simulink model "Converter4"  (R2025a)
settings: Solver=VariableStepAuto  StartTime=0.0  StopTime=10  MaxStep=1e-3  RelTol=1e-3  EnableMultiTasking=on
PreLoadFcn:
  | DualActiveBridgeConverterData
values from neighbouring files (symbols this model uses):
  C_HV = 100e-6    (= 0.0001)    [Converter_Data.m]
  C_LV = 2000e-6    (= 0.002)    [Converter_Data.m]
  Cs_FET = inf    [Converter_Data.m]
  Fsw = 100e3    (= 100000)    [Converter_Data.m]
  Ki_Ireg = 1    [Converter_Data.m]
  Kp_Ireg = 0.01    [Converter_Data.m]
  L_Inductor = 15e-6    (= 1.5e-05)    [Converter_Data.m]
  Lm_Tr = 720e-6    (= 0.00072)    [Converter_Data.m]
  Lprim_Tr = 17e-6    (= 1.7e-05)    [Converter_Data.m]
  Lsec_Tr = 0    [Converter_Data.m]
  N_Tr = 16    [Converter_Data.m]
  Pnom = 100e3    (= 100000)    [Converter_Data.m]
  R_DCsrc1 = 10e-4    (= 0.001)    [Converter_Data.m]
  R_DCsrc2 = 10e-4    (= 0.001)    [Converter_Data.m]
  R_Inductor = 16e-3    (= 0.016)    [Converter_Data.m]
  RC_HV = 1e-6    (= 1e-06)    [Converter_Data.m]
  RC_LV = 1e-6    (= 1e-06)    [Converter_Data.m]
  Rm_Tr = 10e3    (= 10000)    [Converter_Data.m]
  Ron_Diode = 10e-3    (= 0.01)    [Converter_Data.m]
  Ron_FET = 16e-3    (= 0.016)    [Converter_Data.m]
  Rprim_Tr = 43e-6    (= 4.3e-05)    [Converter_Data.m]
  Rs_FET = 1e6    (= 1000000)    [Converter_Data.m]
  Rsec_Tr = 1e-6    (= 1e-06)    [Converter_Data.m]
  Ts = 1e-6    (= 1e-06)    [Converter_Data.m]
  Ts_Control = Ts    (= 1e-06)    [Converter_Data.m]
  Vf_Diode = 4.2    [Converter_Data.m]
  Vnom_HV = 800    [Converter_Data.m]
  Vnom_LV = 48    [Converter_Data.m]
undefined symbols (not defined in the file or in its folder): DiscIntNeverNeededParam, Ts_Power
libraries: simulink x10, spsDiodeLib x8, spsIdealSwitchLib x8, spsSeriesRLCBranchLib x5, spsVoltageMeasurementLib x4, spsCurrentMeasurementLib x3, spsDCVoltageSourceLib x2, spsMeanLib x2, simulink_extras x2, spsSawtoothGeneratorLib x2, spsFirstOrderFilterLib x1, slpidlib x1
settings Model: ExtModeAutoUpdateStatusClock=off  Creator=The MathWorks, Inc.
settings SolverCC: AlgebraicLoopSolver=TrustRegion  AutoInsertRateTranBlk=on
settings DataIOCC: LimitDataPoints=on  SaveFormat=Array  SaveOutput=off  DSMLogging=off  SaveTime=off  ReturnWorkspaceOutputs=off
settings OptimizationCC: LifeSpan=inf
settings DebuggingCC: SaveWithParameterizedLinksMsg=none  UnderspecifiedInitializationDetection=Classic  MergeDetectMultiDrivingBlocksExec=none  SolverPrmCheckMsg=warning  FcnCallInpInsideContextMsg=warning  UnconnectedInputMsg=warning  UnconnectedOutputMsg=warning  UnconnectedLineMsg=warning  StateNameClashWarn=warning  SubsystemReferenceDiagnosticForUnitTest=warning  SFUnexpectedBacktrackingDiag=warning  SFNoUnconditionalDefaultTransitionDiag=warning  SFExecutionAtInitializationDiag=none  ArithmeticOperatorsInVariantConditions=warning
settings HardwareCC: ProdBitPerPointer=32.0  ProdBitPerSizeT=32.0  ProdBitPerPtrDiffT=32.0  ProdLargestAtomicFloat=None  ProdIntDivRoundTo=Undefined  ProdEndianess=Unspecified  ProdWordSize=32.0  ProdHWDeviceType=32-bit Generic  TargetHWDeviceType=32-bit Generic
settings ModelReferenceCC: EnableRefExpFcnMdlSchedulingChecks=on  PropagateSignalLabelsOutOfModel=off
settings SFSimCC: SimUseLocalCustomCode=off  CustomCodeUndefinedFunction=UseInterfaceOnly
settings RTWCC: RTWUseLocalCustomCode=off  GPUComputeCapability=3.5  DLArmComputeVersion=19.05
settings CodeAppCC: StateflowObjectComments=on
settings GRTTargetCC: TargetFcnLib=ansi_tfl_tmw.mat  TargetLangStandard=C89/C90 (ANSI)  CombineOutputUpdateFcns=off  GRTInterface=on
settings ConfigComp: CovMetricSettings=dw  CovSaveCumulativeToWorkspaceVar=on  CovSaveSingleToWorkspaceVar=on  CovExternalEMLEnable=off  CovSFcnEnable=off

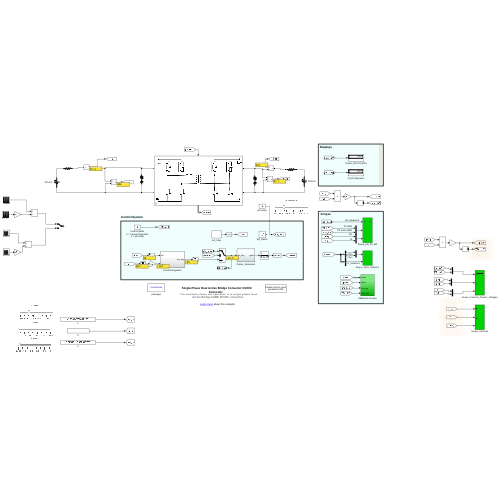
[thumbnail: Simulink's stored preview of the top-level diagram]
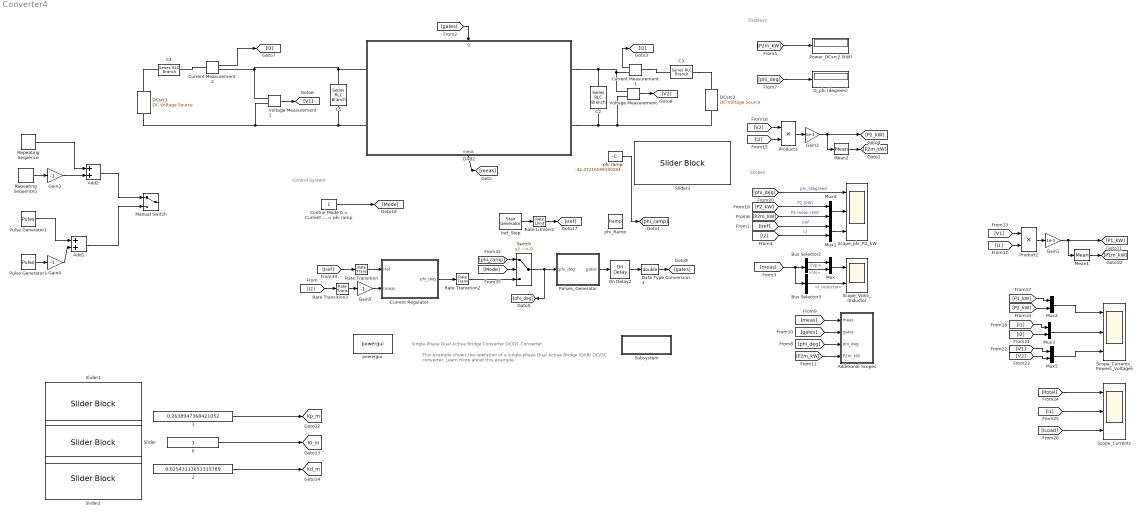
== system Converter4 ==
  note: Single-Phase Dual Active Bridge Converter DC/DC Converter
  note: This example shows the operation of a single-phase Dual Active Bridge (DAB) DC/DC converter.
      |
      | Learn more about this example.
  note: Displays
  note: Scopes
  note: Control System
  0 : Constant
  1 : Constant  Value=0.2638947368421052
  2 : Constant  Value=0.02543113651315789
  Add1 : Sum
  Add2 : Sum
  Additional Scopes : Subsystem
  Bus Selector2 : BusSelector  OutputSignals=Vp,Vs
  Bus Selector3 : BusSelector  OutputSignals=I_Inductor
  C2 : spsSeriesRLCBranchLib/Series RLC Branch  LConnTagsString=__new0  RConnTagsString=__new0  BranchType=RC  Resistance=RC_LV  Inductance=1  SetiL0=off  InitialCurrent=0  Capacitance=C_LV  Setx0=off  InitialVoltage=0  Measurements=None
  C3 : spsSeriesRLCBranchLib/Series RLC Branch  LConnTagsString=__new0  RConnTagsString=__new0  BranchType=R  Resistance=R_DCsrc2  Inductance=100e-6  SetiL0=off  InitialCurrent=0  Capacitance=1  Setx0=off  InitialVoltage=0  Measurements=None
  C4 : spsSeriesRLCBranchLib/Series RLC Branch  LConnTagsString=__new0  RConnTagsString=__new0  BranchType=R  Resistance=R_DCsrc1  Inductance=1  SetiL0=off  InitialCurrent=0  Capacitance=1  Setx0=off  InitialVoltage=0  Measurements=None
  C5 : spsSeriesRLCBranchLib/Series RLC Branch  LConnTagsString=__new0  RConnTagsString=__new0  BranchType=RC  Resistance=RC_HV  Inductance=1  SetiL0=off  InitialCurrent=0  Capacitance=C_HV  Setx0=off  InitialVoltage=0  Measurements=None
  Control Mode 0 = Current Regulator 1 = phi ramp : Constant
  Current Measurement1 : spsCurrentMeasurementLib/Current Measurement  PhasorSimulation=off  OutputType=Complex  PSBequivalent=0
  Current Measurement2 : spsCurrentMeasurementLib/Current Measurement  PhasorSimulation=off  OutputType=Complex  PSBequivalent=0
  Current Regulator : Subsystem
  DAB2 : Subsystem  mask(Single-phase, Dual-Active Bridge DC/DC Converter){Ron_FET=Ron_FET, RsCs_FET=[Rs_FET, Cs_FET], Ron_Diode=Ron_Diode, Vf_Diode=Vf_Diode, RL_Inductor=[R_Inductor, L_Inductor], Param1_Tr=[Pnom, Fsw], Param2_Tr=[Vnom_HV, Rprim_Tr, Lprim_Tr], Param3_Tr=[Vnom_HV/N_Tr, Rsec_Tr, Lsec_Tr], Param4_Tr=[Rm_Tr, Lm_Tr]}
      mask prompts: Ron_FET "Ron FET"; RsCs_FET "FET snubber: [Rs (ohm)  Cs (F)]"; RL_Inductor "Coupling inductor [ R (ohms)   L (H)]"; Param1_Tr "Nominal power and frequency [Pn(VA) fn(Hz)]:"; Param2_Tr "Winding 1 parameters [V1(Vrms) R1(ohm) L1(H)]:"; Param3_Tr "Winding 2 parameters [V2(Vrms) R2(ohm) L2(H)]:"; Param4_Tr "Magnetization resistance and inductance [Rm(ohm) Lm(H)]:"
      mask init:
      | Rs_FET=RsCs_FET(1);
      | Cs_FET=RsCs_FET(2);
      | R_Inductor=RL_Inductor(1);
      | L_Inductor=RL_Inductor(2);
      settings: PortSchema="{\"entries\":[{\"content\":{\"sides\":[{\"content\":{\"connectorIds\":[\"LConn1\",\"LConn2\"]},\"type\":\"ConnectorPlacement.EquallySpacedRectSide\",\"uuid\":\"9324ea44-499c-4ecb-9e49-362befe9c555\"},{\"content\":{\"connectorIds\":[\"RConn1\",\"RConn2\"],\"side\":\"RIGHT\"},\"type\":\"ConnectorPlacement.EquallySpacedRectSide\",\"uuid\":\"1d2d188e-4a2f-457a-9d2e-cac68811a3aa\"},{\"content\":{\"connectorIds\":[\"In1\"],\"side\":\"TOP\"},\"type\":\"ConnectorPlacement.EquallySpacedRectSide\",\"uuid\":\"7f41b21e-a624-46b0-bf38-abdafc8e74d0\"},{\"content\":{\"connectorIds\":[\"Out1\"],\"side\":\"BOTTOM\"},\"type\":\"ConnectorPlacement.EquallySpacedRectSide\",\"uuid\":\"ef27d855-3875-49de-80dc-d9576eabadca\"}]},\"type\":\"ConnectorPlacement.EquallySpacedConnector\",\"uuid\":\"30393c4b-568d-4140-9cdd-d3267fa7bc9d\"}],\"packageUris\":[\"http://schema.mathworks.com/mf0/Connector/R2020b\"],\"version\":\"1.0\"}"
      mask Display: image('DAB_FB1_1.png');
  DCsrc1 : spsDCVoltageSourceLib/DC Voltage Source  Amplitude=Vnom_HV  Measurements=None
  DCsrc2 : spsDCVoltageSourceLib/DC Voltage Source  Amplitude=Vnom_LV  Measurements=None
  D_phi (degrees) : Display
      settings: Format=bank  Decimation=100
  Data Type Conversion1 : DataTypeConversion  OutDataTypeStr=double  SaturateOnIntegerOverflow=off  RndMeth=Floor
  Gain1 : Gain  Gain=1e-3
  Gain2 : Gain  Gain=1e-3
  Gain3 : Gain  Gain=-1
  Gain4 : Gain  Gain=-1
  Gain5 : Gain  Gain=-1
  Iref_Step : spsStairGeneratorLib/Stair Generator  t=[0, 0.01]  e=[0 40]  Ts=0
  Manual Switch : ManualSwitch
  Mean1 : spsMeanLib/Mean  Freq=Fsw  Vinit=0  Ts=0
  Mean2 : spsMeanLib/Mean  Freq=Fsw  Vinit=0  Ts=0
  Mux{,1..5} (6 alike) : Mux  Inputs=2
  On Delay2 : spsOnDelayLib/On Delay  DelayType=On delay  delay=DT  ic=0  Ts=0
  Power_DCsrc2 (kW) : Display
      settings: Format=bank  Decimation=100
  Product1 : Product
  Product2 : Product
  Pulse Generator1 : DiscretePulseGenerator  PulseType=Time based  Amplitude=50  Period=0.5  PulseWidth=50
  Pulse Generator3 : DiscretePulseGenerator  PulseType=Time based  Amplitude=50  Period=0.5  PulseWidth=50  PhaseDelay=0.25
  Pulses_Generator : Subsystem
  Rate Limiter2 : RateLimiter  RisingSlewLimit=3000  FallingSlewLimit=-3000  SampleTimeMode=inherited
  Rate Transition : RateTransition  OutPortSampleTime=Ts_Control
  Rate Transition2 : RateTransition  OutPortSampleTime=0
  Rate Transition3 : RateTransition  OutPortSampleTime=Ts_Control
  Repeating Sequence : simulink/Sources/Repeating Sequence  rep_seq_t=[0 0.25 0.5 0.75 1 ]  rep_seq_y=[0 20 0 0 0]
  Repeating Sequence1 : simulink/Sources/Repeating Sequence  rep_seq_t=[0 0.25 0.5 0.75 1 ]  rep_seq_y=[0 0 0 20 0]
  Scope_Currents : Scope  NumInputPorts=3
      settings: ActiveDisplayYMinimum=-4.638762576316565  ActiveDisplayYMaximum=13.65424069845692  DataLoggingDecimation=Scope_Decimation  DataLoggingVariableName=ScopeData_phi_P2_kW2
  Scope_Currents_Powers_Voltages : Scope  NumInputPorts=3
      settings: ActiveDisplayYMinimum=-39.981992258178039  ActiveDisplayYMaximum=11.99262168602651  DataLoggingDecimation=Scope_Decimation  DataLoggingVariableName=ScopeData_phi_P2_kW1
  Scope_VpVs_IInductor : Scope  NumInputPorts=2
      settings: TimeSpan=0.0001  ActiveDisplayYMinimum=-1012.21746  ActiveDisplayYMaximum=1013.17909  DataLoggingDecimation=Scope_Decimation  DataLoggingVariableName=Scope_VpVs_IInductor
  Scope_phi_P2_kW : Scope  NumInputPorts=3
      settings: ActiveDisplayYMinimum=-12.508064705091812  ActiveDisplayYMaximum=29.1675627450102  DataLoggingDecimation=Scope_Decimation  DataLoggingVariableName=ScopeData_phi_P2_kW
  Slider : SliderBlock  ScaleMin=1  ScaleMax=1000
  Slider1 : SliderBlock  ScaleMin=0.001  ScaleMax=1
  Slider2 : SliderBlock  ScaleMin=1e-06  ScaleMax=1
  Slider3 : SliderBlock  ScaleMin=-90  ScaleMax=90
  Subsystem : Subsystem
      settings: OpenFcn=open('DualActiveBridgeConverterData')
      mask Display: disp('Double-click to open\nparameters file')
  Switch : Switch  Criteria=u2 ~= 0  SaturateOnIntegerOverflow=off  InputSameDT=off
  Voltage Measurement : spsVoltageMeasurementLib/Voltage Measurement  PhasorSimulation=off  OutputType=Complex  PSBequivalent=0
  Voltage Measurement1 : spsVoltageMeasurementLib/Voltage Measurement  PhasorSimulation=off  OutputType=Complex  PSBequivalent=0
  phi ramp : Constant  Value=-42.47216599190284
  phi_Ramp : simulink/Sources/Ramp  slope=200*1/0.04  start=0  InitialOutput=-100
  powergui : spspowerguiLib/powergui  Priority=1  SimulationMode=Continuous  SampleTime=Ts_Power  frequency=60  Iterations=50  frequencyindice=0  Pbase=100e6  ErrMax=1e-4  UnitsV=kV  UnitsW=MW  buscounter=0  FunctionMessages=off  echomessages=off  EnableUseOfTLC=off  CurrentSourceSwitches=on  DisableSnubberDevices=off  DisableRonSwitches=off  DisableVfSwitches=off  DisplayEquations=off  AutomaticDiscreteSolvers=off  SolverType=Tustin/Backward Euler (TBE)  Interpol=off  ExternalGateDelay=off  methode=off  Ts=10  x0status=blocks  SPID=on  SwTol=0  HookPort=off  NonlinearTolerance=1e-4  nMaxIteration=100  ContinueOnMaxIteration=off  RestoreLinks=warning  ResistiveCurrentMeasurement=off  Frange=[0:2:500]  Ylog=off  Xlog=on  ShowGrid=off  save=off  variable=ZData  structure=0  ZoomFFT=off  StartTime=0.0  cycles=1  DisplayStyle=1  fundamental=60  FreqAxis=off  MaxFrequency=1000  frequencyindicesteady=1  RmsSteady=1  display=off
  tag scope: Kd_m=global, Ki_m=global, Kp_m=global
  wires:
  Mean1/1 -> [P1m_kW]
  Gain1/1 -> Mean1/1, [P1_kW]
  [I1] -> Product2/2
  Product2/1 -> Gain1/1
  [V1] -> Product2/1
  [P1_kW] -> Mux2/1
  [P2_kW] -> Mux2/2
  [I1] -> Mux3/1
  [I2] -> Mux3/2
  [V1] -> Mux5/1
  [V2] -> Mux5/2
  Mux2/1 -> Scope_Currents_Powers_Voltages/1
  Mux3/1 -> Scope_Currents_Powers_Voltages/2
  Mux5/1 -> Scope_Currents_Powers_Voltages/3
  Add2/1 -> Manual Switch/1
  Pulse Generator1/1 -> Add1/1
  Gain4/1 -> Add1/2
  Repeating Sequence/1 -> Add2/1
  Pulse Generator3/1 -> Gain4/1
  Gain3/1 -> Add2/2
  Repeating Sequence1/1 -> Gain3/1
  Add1/1 -> Manual Switch/2
  [Itotal] -> Scope_Currents/1
  [I1] -> Scope_Currents/2
  [ILoad] -> Scope_Currents/3
  Product1/1 -> Gain2/1
  Rate Limiter2/1 -> [Iref]
  Pulses_Generator/1(gates) -> On Delay2/1
  Bus Selector2/1 -> Mux/1  "<Vp>"
  [phi_deg] -> Additional Scopes/3(phi_deg)
  [meas] -> Bus Selector3/1, Bus Selector2/1
  Switch/1 -> [phi_deg], Pulses_Generator/1(phi_deg)
  Mux4/1 -> Scope_phi_P2_kW/2
  [phi_deg] -> D_phi (degrees)/1
  Data Type Conversion1/1 -> [gates]
  [P2m_kW] -> Additional Scopes/4(P2m_kW)
  [phi_deg] -> Scope_phi_P2_kW/1  "phi_(degrees)"
  [I2] -> Product1/2
  [Iref] -> Mux1/1  "Iref"
  On Delay2/1 -> Data Type Conversion1/1
  DAB2/1(meas) -> [meas]
  Mux/1 -> Scope_VpVs_IInductor/1
  [P2m_kW] -> Power_DCsrc2 (kW)/1
  Iref_Step/1 -> Rate Limiter2/1
  Current Measurement1/1 -> [I2]
  Gain5/1 -> Current Regulator/2(Imeas)
  Rate Transition2/1 -> Switch/3
  Bus Selector3/1 -> Scope_VpVs_IInductor/2  "<I_Inductor>"
  Bus Selector2/2 -> Mux/2  "<Vs>"
  [V2] -> Product1/1
  [Mode] -> Switch/2
  [Iref] -> Rate Transition/1
  Control Mode 0 = Current Regulator 1 = phi ramp/1 -> [Mode]
  [gates] -> DAB2/1(g)
  Mux1/1 -> Scope_phi_P2_kW/3
  Rate Transition/1 -> Current Regulator/1(Iref)
  phi ramp/1 -> [phi_ramp]
  [I2] -> Rate Transition3/1
  [P2_kW] -> Mux4/1  "P2 (kW)"
  Voltage Measurement/1 -> [V2]
  [gates] -> Additional Scopes/2(gates)
  [phi_ramp] -> Switch/1
  [P2m_kW] -> Mux4/2  "P2 mean (kW)"
  [I2] -> Mux1/2  "I2"
  Gain2/1 -> Mean2/1, [P2_kW]
  [meas] -> Additional Scopes/1(meas)
  Current Regulator/1(phi_deg) -> Rate Transition2/1
  Mean2/1 -> [P2m_kW]
  Voltage Measurement1/1 -> [V1]
  Current Measurement2/1 -> [I1]
  1/1 -> [Kp_m]
  0/1 -> [Ki_m]
  2/1 -> [Kd_m]
  Rate Transition3/1 -> Gain5/1
  connections:
  DCsrc2/LConn1 -- C2/RConn1 -- DAB2/RConn2 -- Voltage Measurement/LConn2
  C5/LConn1 -- Current Measurement2/RConn1 -- Voltage Measurement1/LConn1 -- DAB2/LConn1
  DAB2/LConn2 -- C5/RConn1 -- Voltage Measurement1/LConn2 -- DCsrc1/LConn1
  C2/LConn1 -- Current Measurement1/RConn1 -- Voltage Measurement/LConn1 -- DAB2/RConn1
  C4/RConn1 -- DCsrc1/RConn1
  C3/LConn1 -- DCsrc2/RConn1
  Current Measurement2/LConn1 -- C4/LConn1
  Current Measurement1/LConn1 -- C3/RConn1

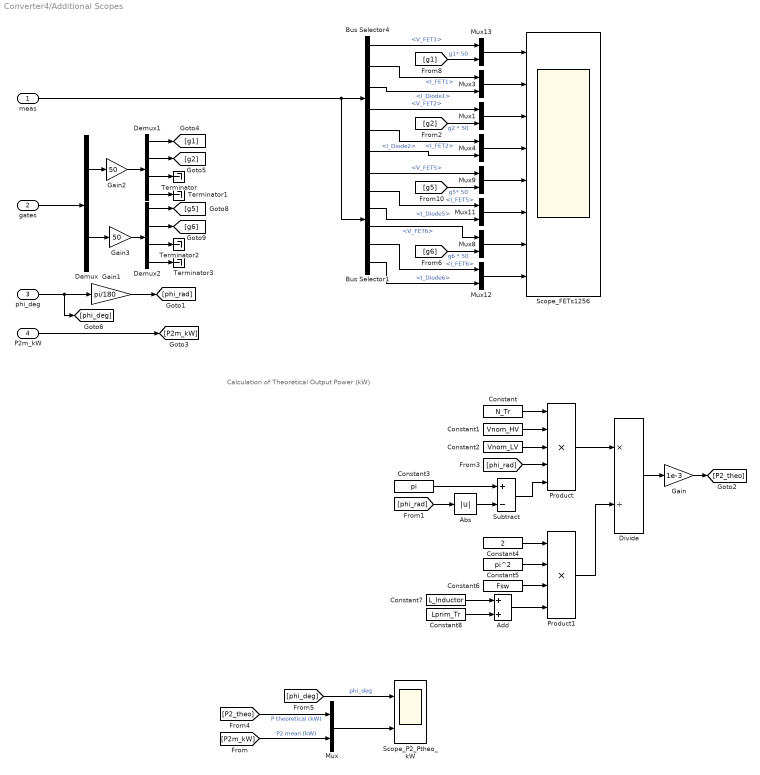
== system Converter4/Additional Scopes ==
  note: Calculation of Theoretical Output Power (kW)
  meas : Inport
  gates : Inport  Port=2
  phi_deg : Inport  Port=3
  P2m_kW : Inport  Port=4
  Abs : Abs  SaturateOnIntegerOverflow=off
  Add : Sum
  Bus Selector1 : BusSelector  OutputSignals=V_FET5,I_FET5,I_Diode5,V_FET6,I_FET6,I_Diode6
  Bus Selector4 : BusSelector  OutputSignals=V_FET1,I_FET1,I_Diode1,V_FET2,I_FET2,I_Diode2
  Constant : Constant  Value=N_Tr
  Constant1 : Constant  Value=Vnom_HV
  Constant2 : Constant  Value=Vnom_LV
  Constant3 : Constant  Value=pi
  Constant4 : Constant  Value=2
  Constant5 : Constant  Value=pi^2
  Constant6 : Constant  Value=Fsw
  Constant7 : Constant  Value=L_Inductor
  Constant8 : Constant  Value=Lprim_Tr
  Demux : Demux  Outputs=[4,4]
  Demux1 : Demux
  Demux2 : Demux
  Divide : Product  Inputs=*/
  Gain : Gain  Gain=1e-3
  Gain1 : Gain  Gain=pi/180
  Gain2 : Gain  Gain=50
  Gain3 : Gain  Gain=50
  Mux{,1,3..4,8..9,11..13} (9 alike) : Mux  Inputs=2
  Product : Product  Inputs=5
  Product1 : Product  Inputs=4
  Scope_FETs1256 : Scope  NumInputPorts=8
      settings: TimeSpan=0.0005  ActiveDisplayYMinimum=-105.52087  ActiveDisplayYMaximum=905.58143  DataLoggingMaxPoints=20000  DataLoggingDecimation=Scope_Decimation  DataLoggingVariableName=ScopeData_FETs1256
  Scope_P2_Ptheo_kW : Scope  NumInputPorts=2
      settings: TimeSpan=0.0005  ActiveDisplayYMinimum=-125  ActiveDisplayYMaximum=125  DataLoggingMaxPoints=20000  DataLoggingDecimation=Scope_Decimation  DataLoggingVariableName=Scope_phi_Ptheo_P2_kW
  Subtract : Sum  Inputs=+-
  Terminator{,1..3} (4 alike) : Terminator
  wires:
  gates/1 -> Demux/1
  Bus Selector4/1 -> Mux13/1  "<V_FET1>"
  [g1] -> Mux13/2  "g1* 50"
  Mux13/1 -> Scope_FETs1256/1
  [g2] -> Mux1/2  "g2 * 50"
  Bus Selector4/4 -> Mux1/1  "<V_FET2>"
  Mux3/1 -> Scope_FETs1256/2
  Bus Selector4/2 -> Mux3/1  "<I_FET1>"
  Bus Selector4/3 -> Mux3/2  "<I_Diode1>"
  Mux1/1 -> Scope_FETs1256/3
  Mux4/1 -> Scope_FETs1256/4
  Bus Selector4/5 -> Mux4/1  "<I_FET2>"
  Bus Selector4/6 -> Mux4/2  "<I_Diode2>"
  Bus Selector1/6 -> Mux12/2  "<I_Diode6>"
  Bus Selector1/5 -> Mux12/1  "<I_FET6>"
  Bus Selector1/3 -> Mux11/2  "<I_Diode5>"
  Bus Selector1/2 -> Mux11/1  "<I_FET5>"
  Bus Selector1/4 -> Mux8/1  "<V_FET6>"
  [g6] -> Mux8/2  "g6 * 50"
  [g5] -> Mux9/2  "g5* 50"
  Bus Selector1/1 -> Mux9/1  "<V_FET5>"
  Demux/1 -> Gain2/1
  Demux/2 -> Gain3/1
  Gain2/1 -> Demux1/1
  Demux1/1 -> [g1]
  Demux1/2 -> [g2]
  Demux1/3 -> Terminator/1
  Demux1/4 -> Terminator1/1
  Gain3/1 -> Demux2/1
  Demux2/1 -> [g5]
  Demux2/2 -> [g6]
  Demux2/3 -> Terminator2/1
  Demux2/4 -> Terminator3/1
  Mux9/1 -> Scope_FETs1256/5
  Mux11/1 -> Scope_FETs1256/6
  Mux8/1 -> Scope_FETs1256/7
  Mux12/1 -> Scope_FETs1256/8
  meas/1 -> Bus Selector1/1, Bus Selector4/1
  phi_deg/1 -> [phi_deg], Gain1/1
  Gain1/1 -> [phi_rad]
  Constant3/1 -> Subtract/1
  [phi_rad] -> Abs/1
  Constant/1 -> Product/1
  Constant1/1 -> Product/2
  Constant2/1 -> Product/3
  Abs/1 -> Subtract/2
  Subtract/1 -> Product/5
  Product/1 -> Divide/1
  Constant4/1 -> Product1/1
  Constant5/1 -> Product1/2
  Constant6/1 -> Product1/3
  Add/1 -> Product1/4
  Constant7/1 -> Add/1
  Constant8/1 -> Add/2
  Product1/1 -> Divide/2
  Divide/1 -> Gain/1
  P2m_kW/1 -> [P2m_kW]
  Gain/1 -> [P2_theo]
  [P2_theo] -> Mux/1  "P theoretical (kW)"
  [P2m_kW] -> Mux/2  "P2 mean (kW)"
  [phi_rad] -> Product/4
  Mux/1 -> Scope_P2_Ptheo_kW/2
  [phi_deg] -> Scope_P2_Ptheo_kW/1  "phi_deg"

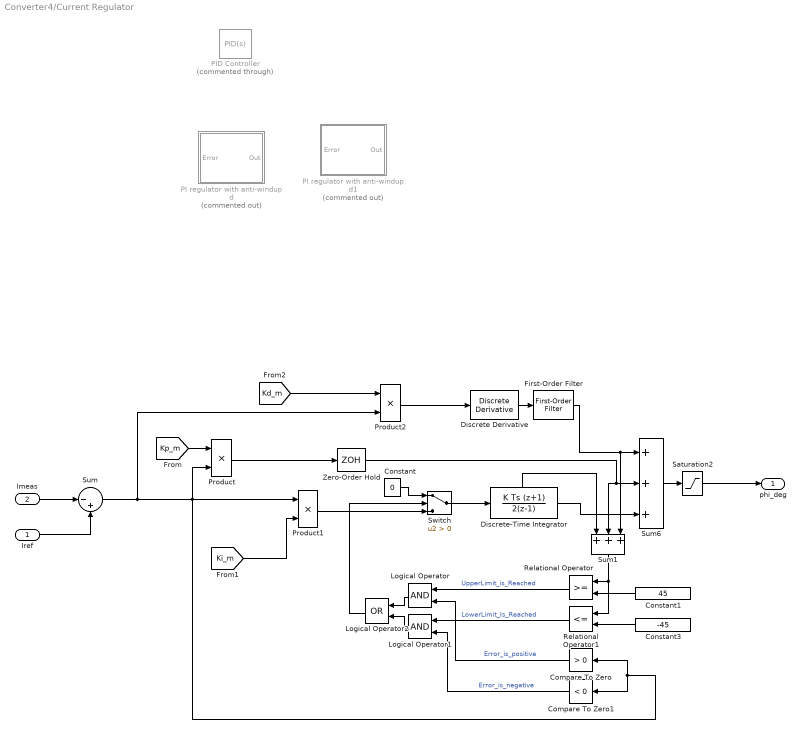
== system Converter4/Current Regulator ==
  Iref : Inport
  Imeas : Inport  Port=2
  Compare To Zero : simulink/Logic and Bit Operations/Compare To Zero  relop=>  OutDataTypeStr=uint8  ZeroCross=off
  Compare To Zero1 : simulink/Logic and Bit Operations/Compare To Zero  relop=<  OutDataTypeStr=uint8  ZeroCross=off
  Constant : Constant  Value=0
  Constant1 : Constant  Value=45
  Constant3 : Constant  Value=-45
  Discrete Derivative : simulink/Discrete/Discrete Derivative  gainval=1.0  ICPrevScaledInput=0.0  OutMin=[]  OutMax=[]  OutDataType=fixdt(1, 16)  OutScaling=2^-10  DoSatur=off
  Discrete-Time Integrator : DiscreteIntegrator  IntegratorMethod=Integration: Trapezoidal  SampleTime=Ts  LimitOutput=on  UpperSaturationLimit=45  LowerSaturationLimit=-45  ShowStatePort=on  ICPrevOutput=DiscIntNeverNeededParam  ICPrevScaledInput=DiscIntNeverNeededParam
  First-Order Filter : spsFirstOrderFilterLib/First-Order Filter  FilterType=Lowpass  Tc=10e-04  Ts=0  Initialize=on  Vac_Init=[0, 0, 60]  Vdc_Init=0  PlotResponse=off  FreqRange="[0,  200,  1]"
  Logical Operator : Logic  AllPortsSameDT=off  OutDataTypeStr=boolean
  Logical Operator1 : Logic  AllPortsSameDT=off  OutDataTypeStr=boolean
  Logical Operator2 : Logic  Operator=OR  AllPortsSameDT=off  OutDataTypeStr=boolean
  PI regulator with anti-windup d : Subsystem  Commented=on  DialogController=POWERSYS.PowerSysDialog  mask(Discrete PI Controller with anti-windup){Kp=Kp_Ireg, Ki=Ki_Ireg, Par_Limits=[500, -500], Init=0, Ts=Ts_Control}
      mask prompts: Kp "Proportional gain (Kp):"; Ki "Integral gain (Ki):"; Par_Limits "Output limits: [ Upper   Lower ]"; Init "Output initial value:"; Ts "Sample time:"
      mask help: This block implements a discrete PI controller with anti-windup.
      mask init:
      | UpperLimit=Par_Limits(1);
      | LowerLimit=Par_Limits(2);
      mask Display: disp('PI');
  PI regulator with anti-windup d1 : Subsystem  Commented=on  DialogController=POWERSYS.PowerSysDialog  mask(Discrete PI Controller with anti-windup){Kp=Kp_Ireg, Ki=Ki_Ireg, Par_Limits=[500, -500], Init=0, Ts=Ts_Control}
      mask prompts: Kp "Proportional gain (Kp):"; Ki "Integral gain (Ki):"; Par_Limits "Output limits: [ Upper   Lower ]"; Init "Output initial value:"; Ts "Sample time:"
      mask help: This block implements a discrete PI controller with anti-windup.
      mask init:
      | UpperLimit=Par_Limits(1);
      | LowerLimit=Par_Limits(2);
      mask Display: disp('PI');
  PID Controller : slpidlib/PID Controller  Commented=through  Controller=PID  Form=Parallel  TimeDomain=Continuous-time  UseExternalTs=off  SampleTime=-1  IntegratorMethod=Forward Euler  FilterMethod=Trapezoidal  ControllerParametersSource=internal  P=0.25724  I=10.926  UseKiTs=off  D=0  UseExternalDerivativeSource=off  N=100  UseFilter=on  TunerSelectOption=Transfer Function Based (PID Tuner App)  InitialConditionSource=internal  InitialConditionForIntegrator=0  InitialConditionForFilter=0  DifferentiatorICPrevScaledInput=0  ExternalReset=none  TrackingMode=off  Kt=1  LimitOutput=on  SatLimitsSource=internal  UpperSaturationLimit=45  LowerSaturationLimit=-45  LinearizeAsGain=on  AntiWindupMode=back-calculation  Kb=0.1  LimitIntegrator=off  UpperIntegratorSaturationLimit=inf  LowerIntegratorSaturationLimit=-inf  POutMin=[]  POutMax=[]  IOutMin=[]  IOutMax=[]  DOutMin=[]  DOutMax=[]  NOutMin=[]  NOutMax=[]  SumOutMin=[]  SumOutMax=[]  SaturationOutMin=[]  SaturationOutMax=[]  PParamMin=[]  PParamMax=[]  IParamMin=[]  IParamMax=[]  DParamMin=[]  DParamMax=[]  NParamMin=[]  NParamMax=[]  KbParamMin=[]  KbParamMax=[]  KtParamMin=[]  KtParamMax=[]  KbOutMin=[]  KbOutMax=[]  KtOutMin=[]  KtOutMax=[]  IntegratorOutMin=[]  IntegratorOutMax=[]  FilterOutMin=[]  FilterOutMax=[]  SumI1OutMin=[]  SumI1OutMax=[]  SumI2OutMin=[]  SumI2OutMax=[]  SumI3OutMin=[]  SumI3OutMax=[]  SumI4OutMin=[]  SumI4OutMax=[]  SumDOutMin=[]  SumDOutMax=[]  DifferentiatorOutMin=[]  DifferentiatorOutMax=[]  FilterDiffOutCoefMin=[]  FilterDiffOutCoefMax=[]  ReciprocalOutMin=[]  ReciprocalOutMax=[]  SumDenOutMin=[]  SumDenOutMax=[]  SumNumOutMin=[]  SumNumOutMax=[]  DivideOutMin=[]  DivideOutMax=[]  UdiffTsProdOutMin=[]  UdiffTsProdOutMax=[]  NTsProdOutMin=[]  NTsProdOutMax=[]  UintegralTsProdOutMin=[]  UintegralTsProdOutMax=[]  UngainTsProdOutMin=[]  UngainTsProdOutMax=[]  ClampingZeroOutDataTypeStr=Inherit: Inherit via back propagation  ClampingZeroOutMin=[]  ClampingZeroOutMax=[]  FilterDenConstantOutDataTypeStr=Inherit: Inherit via back propagation  FilterDenConstantOutMin=[]  FilterDenConstantOutMax=[]  PCopyOutDataTypeStr=Inherit: Inherit via back propagation  PCopyOutMin=[]  PCopyOutMax=[]  NCopyOutDataTypeStr=Inherit: Inherit via back propagation  NCopyOutMin=[]  NCopyOutMax=[]  IntegratorContinuousStateAttributes=''  IntegratorStateMustResolveToSignalObject=off  IntegratorRTWStateStorageClass=Auto  FilterContinuousStateAttributes=''  FilterStateMustResolveToSignalObject=off  FilterRTWStateStorageClass=Auto  ParallelPVariant=InternalParameters  IdealPVariant=Disabled  IVariant=InternalParameters  DVariant=InternalParameters  IntegratorVariant=Continuous  SatVariant=Enabled  AWVariant=BackCalculation  PCopyVariant=Disabled  TRVariant=Disabled  FdbkBlocksVariant=Forward  IdealPFdbkVariant=Disabled  SatFdbkVariant=Disabled  DerivativeFilterVariant=ContFilter  NVariant=InternalParameters  NCopyVariant=Disabled  FilterICVariant=InternalICsFilter  IntegratorICVariant=InternalICs  ExternalResetVariant=Disabled  TRSumVariant=Passthrough  SumFdbkVariant=Disabled  SumVariant=Sum_PID  TsampFilterVariant=InternalTs  TsampNgainVariant=Passthrough  TsampIntegralVariant=Disabled_SignalSpec  ExternalSaturationOutDataTypeStr=Inherit: Same as second input  DerivativeSourceVariant=ErrorSignal  PreIntVariant=InternalPreInt
  Product : Product
  Product1 : Product
  Product2 : Product
  Relational Operator : RelationalOperator  OutDataTypeStr=boolean  InputSameDT=off
  Relational Operator1 : RelationalOperator  Operator=<=  OutDataTypeStr=boolean  InputSameDT=off
  Saturation2 : Saturate  UpperLimit=45  LowerLimit=-45  SampleTime=Ts
  Sum : Sum  Inputs=|-+
  Sum1 : Sum  Inputs=+++  InputSameDT=on  SaturateOnIntegerOverflow=on  SampleTime=Ts  OutDataTypeStr=Inherit: Same as first input
  Sum6 : Sum  Inputs=+++  InputSameDT=on  SaturateOnIntegerOverflow=on  SampleTime=Ts  OutDataTypeStr=Inherit: Same as first input
  Switch : Switch  Criteria=u2 > Threshold  SaturateOnIntegerOverflow=off  InputSameDT=off
  Zero-Order Hold : ZeroOrderHold  SampleTime=Ts
  phi_deg : Outport
  wires:
  Imeas/1 -> Sum/1
  Iref/1 -> Sum/2
  Saturation2/1 -> phi_deg/1
  Constant1/1 -> Relational Operator/2
  Discrete-Time Integrator/State -> Sum1/1
  Discrete-Time Integrator/1 -> Sum6/3
  Constant3/1 -> Relational Operator1/2
  Switch/1 -> Discrete-Time Integrator/1
  Constant/1 -> Switch/1
  Compare To Zero1/1 -> Logical Operator1/2  "Error_is_negative"
  Relational Operator/1 -> Logical Operator/1  "UpperLimit_is_Reached"
  Logical Operator2/1 -> Switch/2
  Sum/1 -> Product2/2, Compare To Zero1/1, Compare To Zero/1, Product/2, Product1/1
  Product/1 -> Zero-Order Hold/1
  [Ki_m] -> Product1/2
  Relational Operator1/1 -> Logical Operator1/1  "LowerLimit_Is_Reached"
  Logical Operator/1 -> Logical Operator2/1
  [Kp_m] -> Product/1
  Product1/1 -> Switch/3
  Logical Operator1/1 -> Logical Operator2/2
  Sum6/1 -> Saturation2/1
  Compare To Zero/1 -> Logical Operator/2  "Error_is_positive"
  Zero-Order Hold/1 -> Sum6/2, Sum1/2
  Sum1/1 -> Relational Operator1/1, Relational Operator/1
  Discrete Derivative/1 -> First-Order Filter/1
  Product2/1 -> Discrete Derivative/1
  [Kd_m] -> Product2/1
  First-Order Filter/1 -> Sum1/3, Sum6/1

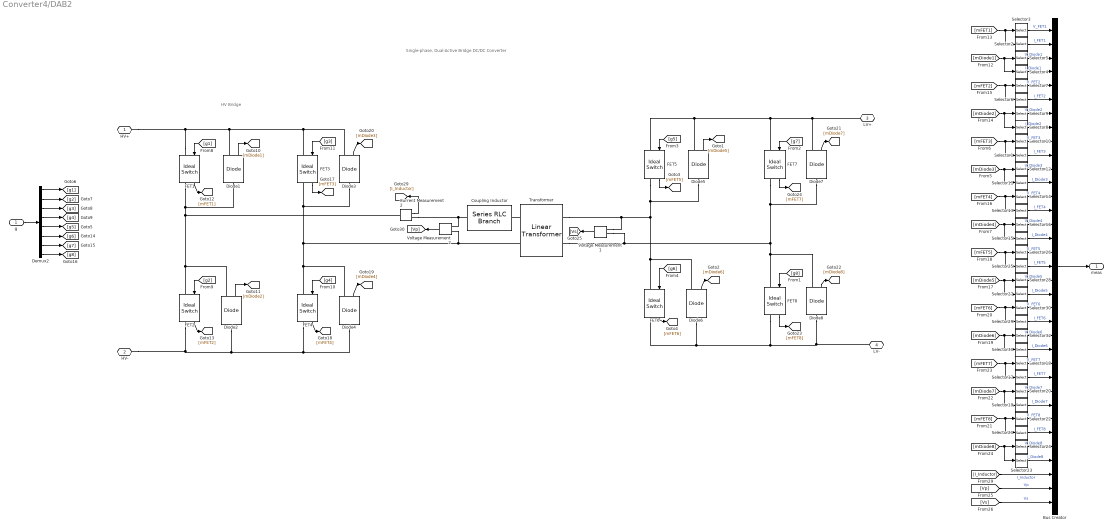
== system Converter4/DAB2 ==
  note: HV Bridge
  note: Single-phase, Dual-Active Bridge
      | DC/DC Converter
  g : Inport  PortDimensions=8
  Bus Creator : BusCreator  Inputs=35
  Coupling Inductor : spsSeriesRLCBranchLib/Series RLC Branch  LConnTagsString=__new0  RConnTagsString=__new0  BranchType=RL  Resistance=R_Inductor  Inductance=L_Inductor  SetiL0=off  InitialCurrent=0  Capacitance=1e-6  Setx0=off  InitialVoltage=0  Measurements=None
  Current Measurement2 : spsCurrentMeasurementLib/Current Measurement  PhasorSimulation=off  OutputType=Complex  PSBequivalent=0
  Demux2 : Demux  Outputs=8
  Diode{1..8} (8 alike) : spsDiodeLib/Diode  Ron=Ron_Diode  Lon=0  Vf=Vf_Diode  IC=0  UseSnubber=0  Rs=inf  Cs=inf  Measurements=on
  FET{1..8} (8 alike) : spsIdealSwitchLib/Ideal Switch  Ron=Ron_FET  Lon=0  IC=0  Rs=Rs_FET  Cs=Cs_FET  Measurements=on
  Selector{1..2,4,6,8,11,13,15,17,19,21,23,25,27,29,31} (16 alike) : Selector  InputPortWidth=2  IndexOptions=Index vector (dialog)  Indices=1  OutputSizes=1
  Selector{3,5,7,9..10,12,14,16,18,20,22,24,26,28,30,32} (16 alike) : Selector  InputPortWidth=2  IndexOptions=Index vector (dialog)  Indices=2  OutputSizes=1
  Transformer : spsLinearTransformerLib/Linear Transformer  UNITS=SI  NominalPower="[ Param1_Tr(1),  Param1_Tr(2)]"  winding1="[ Param2_Tr(1),  Param2_Tr(2), Param2_Tr(3)]"  winding2="[ Param3_Tr(1),  Param3_Tr(2), Param3_Tr(3)]"  ThreeWindings=off  winding3=[3.15e+05 0.7938 0.084225]  RmLm="[ Param4_Tr(1),  Param4_Tr(2)]"  Measurements=None  DataType=on
  Voltage Measurement1 : spsVoltageMeasurementLib/Voltage Measurement  PhasorSimulation=off  OutputType=Complex  PSBequivalent=0
  Voltage Measurement2 : spsVoltageMeasurementLib/Voltage Measurement  PhasorSimulation=off  OutputType=Complex  PSBequivalent=0
  HV+ : PMIOPort  Side=Left
  HV- : PMIOPort  Port=2  Side=Left
  LV+ : PMIOPort  Port=3  Side=Right
  LV- : PMIOPort  Port=4  Side=Right
  meas : Outport  PortDimensions=35
  wires:
  Voltage Measurement2/1 -> [Vp]
  Demux2/8 -> [g8]
  Selector20/1 -> Bus Creator/27  "V_Diode7"
  Selector21/1 -> Bus Creator/30  "I_FET8"
  Selector22/1 -> Bus Creator/29  "V_FET8"
  Selector24/1 -> Bus Creator/31  "V_Diode8"
  [mDiode5] -> Selector27/1, Selector28/1
  Selector27/1 -> Bus Creator/20  "I_Diode5"
  [mFET6] -> Selector30/1, Selector29/1
  Selector23/1 -> Bus Creator/32  "I_Diode8"
  Selector32/1 -> Bus Creator/23  "V_Diode6"
  Selector26/1 -> Bus Creator/17  "V_FET5"
  Selector28/1 -> Bus Creator/19  "V_Diode5"
  Selector25/1 -> Bus Creator/18  "I_FET5"
  [mFET5] -> Selector25/1, Selector26/1
  FET3/1 -> [mFET3]
  Diode4/1 -> [mDiode4]
  FET4/1 -> [mFET4]
  Selector19/1 -> Bus Creator/28  "I_Diode7"
  FET7/1 -> [mFET7]
  Selector5/1 -> Bus Creator/3  "V_Diode1"
  [mDiode2] -> Selector8/1, Selector9/1
  [g4] -> FET4/1
  Selector4/1 -> Bus Creator/4  "I_Diode1"
  [mFET4] -> Selector14/1, Selector13/1
  Diode2/1 -> [mDiode2]
  Demux2/1 -> [g1]
  FET1/1 -> [mFET1]
  Selector18/1 -> Bus Creator/25  "V_FET7"
  Selector3/1 -> Bus Creator/1  "V_FET1"
  [mFET8] -> Selector21/1, Selector22/1
  FET2/1 -> [mFET2]
  [mDiode4] -> Selector16/1, Selector15/1
  [g1] -> FET1/1
  [g3] -> FET3/1
  Demux2/4 -> [g4]
  [mFET1] -> Selector3/1, Selector2/1
  Diode1/1 -> [mDiode1]
  Demux2/2 -> [g2]
  Diode6/1 -> [mDiode6]
  Demux2/3 -> [g3]
  Diode5/1 -> [mDiode5]
  [mDiode1] -> Selector5/1, Selector4/1
  Diode3/1 -> [mDiode3]
  Demux2/7 -> [g7]
  Selector6/1 -> Bus Creator/6  "I_FET2"
  Selector2/1 -> Bus Creator/2  "I_FET1"
  [mDiode3] -> Selector11/1, Selector12/1
  Selector13/1 -> Bus Creator/14  "I_FET4"
  Selector10/1 -> Bus Creator/9  "V_FET3"
  [mFET3] -> Selector1/1, Selector10/1
  Selector15/1 -> Bus Creator/16  "I_Diode4"
  Selector16/1 -> Bus Creator/15  "V_Diode4"
  Selector14/1 -> Bus Creator/13  "V_FET4"
  Selector30/1 -> Bus Creator/21  "V_FET6"
  [g7] -> FET7/1
  Demux2/6 -> [g6]
  [g8] -> FET8/1
  Selector9/1 -> Bus Creator/7  "V_Diode2"
  [g2] -> FET2/1
  FET6/1 -> [mFET6]
  Diode7/1 -> [mDiode7]
  [mDiode7] -> Selector20/1, Selector19/1
  Selector11/1 -> Bus Creator/12  "I_Diode3"
  Selector29/1 -> Bus Creator/22  "I_FET6"
  [mFET2] -> Selector6/1, Selector7/1
  [mDiode8] -> Selector23/1, Selector24/1
  Diode8/1 -> [mDiode8]
  FET5/1 -> [mFET5]
  Selector17/1 -> Bus Creator/26  "I_FET7"
  Selector12/1 -> Bus Creator/11  "V_Diode3"
  Current Measurement2/1 -> [I_Inductor]
  Selector1/1 -> Bus Creator/10  "I_FET3"
  Demux2/5 -> [g5]
  Selector31/1 -> Bus Creator/24  "I_Diode6"
  [mFET7] -> Selector18/1, Selector17/1
  Selector8/1 -> Bus Creator/8  "I_Diode2"
  [g5] -> FET5/1
  Selector7/1 -> Bus Creator/5  "V_FET2"
  FET8/1 -> [mFET8]
  [mDiode6] -> Selector32/1, Selector31/1
  [g6] -> FET6/1
  g/1 -> Demux2/1
  Bus Creator/1 -> meas/1
  Voltage Measurement1/1 -> [Vs]
  [I_Inductor] -> Bus Creator/33  "I_Inductor"
  [Vp] -> Bus Creator/34  "Vp"
  [Vs] -> Bus Creator/35  "Vs"
  connections:
  FET7/LConn1 -- LV+/RConn1 -- Diode7/RConn1 -- Diode5/RConn1 -- FET5/LConn1
  FET1/LConn1 -- HV+/RConn1 -- Diode3/RConn1 -- FET3/LConn1 -- Diode1/RConn1
  FET2/RConn1 -- HV-/RConn1 -- FET4/RConn1 -- Diode4/LConn1 -- Diode2/LConn1
  Diode2/RConn1 -- Current Measurement2/LConn1 -- Diode1/LConn1 -- FET1/RConn1 -- FET2/LConn1
  Diode4/RConn1 -- FET4/LConn1 -- Transformer/LConn2 -- Voltage Measurement2/LConn2 -- FET3/RConn1 -- Diode3/LConn1
  FET6/RConn1 -- Diode6/LConn1 -- LV-/RConn1 -- Diode8/LConn1 -- FET8/RConn1
  FET7/RConn1 -- Voltage Measurement1/LConn2 -- Transformer/RConn2 -- FET8/LConn1 -- Diode8/RConn1 -- Diode7/LConn1
  FET6/LConn1 -- Voltage Measurement1/LConn1 -- Transformer/RConn1 -- Diode5/LConn1 -- FET5/RConn1 -- Diode6/RConn1
  Current Measurement2/RConn1 -- Voltage Measurement2/LConn1 -- Coupling Inductor/LConn1
  Transformer/LConn1 -- Coupling Inductor/RConn1

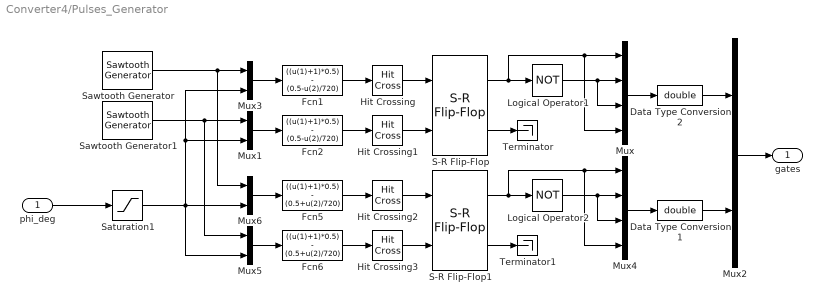
== system Converter4/Pulses_Generator ==
  phi_deg : Inport
  Data Type Conversion1 : DataTypeConversion  OutDataTypeStr=double  SaturateOnIntegerOverflow=off  RndMeth=Floor
  Data Type Conversion2 : DataTypeConversion  OutDataTypeStr=double  SaturateOnIntegerOverflow=off  RndMeth=Floor
  Fcn1 : Fcn  Expr=((u(1)+1)*0.5) - (0.5-u(2)/720)
  Fcn2 : Fcn  Expr=((u(1)+1)*0.5) - (0.5-u(2)/720)
  Fcn5 : Fcn  Expr=((u(1)+1)*0.5) - (0.5+u(2)/720)
  Fcn6 : Fcn  Expr=((u(1)+1)*0.5) - (0.5+u(2)/720)
  Hit Crossing{,1..3} (4 alike) : HitCross  HitCrossingDirection=rising
  Logical Operator1 : Logic  Operator=NOT  AllPortsSameDT=off  OutDataTypeStr=boolean
  Logical Operator2 : Logic  Operator=NOT  AllPortsSameDT=off  OutDataTypeStr=boolean
  Mux : Mux
  Mux{1,3,5..6} (4 alike) : Mux  Inputs=2
  Mux2 : Mux  Inputs=[4,4]
  Mux4 : Mux
  S-R Flip-Flop : simulink_extras/Flip Flops/S-R Flip-Flop  initial_condition=0
  S-R Flip-Flop1 : simulink_extras/Flip Flops/S-R Flip-Flop  initial_condition=0
  Saturation1 : Saturate  UpperLimit=180  LowerLimit=-180
  Sawtooth Generator : spsSawtoothGeneratorLib/Sawtooth Generator  Freq=Fsw  Phase=0  Ts=0
  Sawtooth Generator1 : spsSawtoothGeneratorLib/Sawtooth Generator  Freq=Fsw  Phase=180  Ts=0
  Terminator : Terminator
  Terminator1 : Terminator
  gates : Outport
  wires:
  Mux2/1 -> gates/1
  Logical Operator1/1 -> Mux/2, Mux/3
  phi_deg/1 -> Saturation1/1
  Sawtooth Generator/1 -> Mux6/1, Mux3/1
  Fcn1/1 -> Hit Crossing/1
  Fcn2/1 -> Hit Crossing1/1
  Hit Crossing/1 -> S-R Flip-Flop/1
  Hit Crossing1/1 -> S-R Flip-Flop/2
  S-R Flip-Flop/1 -> Mux/4, Mux/1, Logical Operator1/1
  S-R Flip-Flop/2 -> Terminator/1
  Mux/1 -> Data Type Conversion2/1
  Data Type Conversion2/1 -> Mux2/1
  Data Type Conversion1/1 -> Mux2/2
  Mux3/1 -> Fcn1/1
  Mux1/1 -> Fcn2/1
  Sawtooth Generator1/1 -> Mux5/1, Mux1/1
  Saturation1/1 -> Mux6/2, Mux5/2, Mux1/2, Mux3/2
  Mux5/1 -> Fcn6/1
  Mux6/1 -> Fcn5/1
  Mux4/1 -> Data Type Conversion1/1
  S-R Flip-Flop1/2 -> Terminator1/1
  S-R Flip-Flop1/1 -> Logical Operator2/1, Mux4/1, Mux4/4
  Hit Crossing3/1 -> S-R Flip-Flop1/2
  Hit Crossing2/1 -> S-R Flip-Flop1/1
  Fcn6/1 -> Hit Crossing3/1
  Fcn5/1 -> Hit Crossing2/1
  Logical Operator2/1 -> Mux4/3, Mux4/2

== system Converter4/Subsystem ==

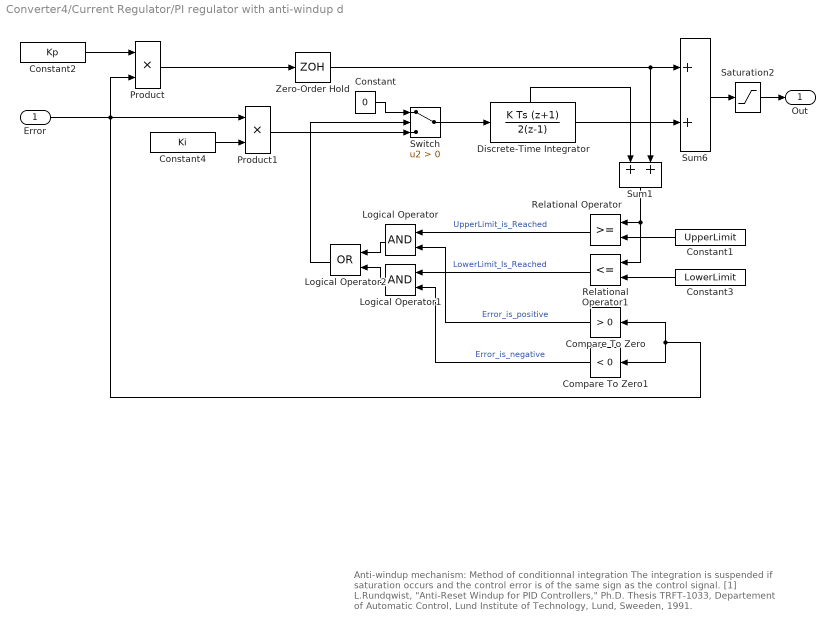
== system Converter4/Current Regulator/PI regulator with anti-windup d ==
  note: Anti-windup mechanism: Method of conditionnal integration
      |
      | The integration is suspended if saturation occurs and the
      | control error is of the same sign as the control signal.
      |
      | [1] L.Rundqwist, "Anti-Reset Windup for PID Controllers," Ph.D. Thesis TRFT-1033,
      | Departement of Automatic Control, Lund Institute of Technology, Lund, Sweeden, 1991.
  Error : Inport  SampleTime=Ts
  Compare To Zero : simulink/Logic and Bit Operations/Compare To Zero  relop=>  OutDataTypeStr=uint8  ZeroCross=off
  Compare To Zero1 : simulink/Logic and Bit Operations/Compare To Zero  relop=<  OutDataTypeStr=uint8  ZeroCross=off
  Constant : Constant  Value=0
  Constant1 : Constant  Value=UpperLimit
  Constant2 : Constant  Value=Kp  SampleTime=Ts
  Constant3 : Constant  Value=LowerLimit
  Constant4 : Constant  Value=Ki  SampleTime=Ts
  Discrete-Time Integrator : DiscreteIntegrator  IntegratorMethod=Integration: Trapezoidal  InitialCondition=Init  SampleTime=Ts  LimitOutput=on  UpperSaturationLimit=UpperLimit  LowerSaturationLimit=LowerLimit  ShowStatePort=on  ICPrevOutput=DiscIntNeverNeededParam  ICPrevScaledInput=DiscIntNeverNeededParam
  Logical Operator : Logic  AllPortsSameDT=off  OutDataTypeStr=boolean
  Logical Operator1 : Logic  AllPortsSameDT=off  OutDataTypeStr=boolean
  Logical Operator2 : Logic  Operator=OR  AllPortsSameDT=off  OutDataTypeStr=boolean
  Product : Product
  Product1 : Product
  Relational Operator : RelationalOperator  OutDataTypeStr=boolean  InputSameDT=off
  Relational Operator1 : RelationalOperator  Operator=<=  OutDataTypeStr=boolean  InputSameDT=off
  Saturation2 : Saturate  UpperLimit=UpperLimit  LowerLimit=LowerLimit  SampleTime=Ts
  Sum1 : Sum  InputSameDT=on  SaturateOnIntegerOverflow=on  SampleTime=Ts  OutDataTypeStr=Inherit: Same as first input
  Sum6 : Sum  InputSameDT=on  SaturateOnIntegerOverflow=on  SampleTime=Ts  OutDataTypeStr=Inherit: Same as first input
  Switch : Switch  Criteria=u2 > Threshold  SaturateOnIntegerOverflow=off  InputSameDT=off
  Zero-Order Hold : ZeroOrderHold  SampleTime=Ts
  Out : Outport  SampleTime=Ts  InitialOutput=0  VectorParamsAs1DForOutWhenUnconnected=off
  wires:
  Constant4/1 -> Product1/2
  Constant/1 -> Switch/1
  Zero-Order Hold/1 -> Sum1/2, Sum6/1
  Discrete-Time Integrator/State -> Sum1/1
  Sum1/1 -> Relational Operator1/1, Relational Operator/1
  Logical Operator2/1 -> Switch/2
  Relational Operator/1 -> Logical Operator/1  "UpperLimit_is_Reached"
  Relational Operator1/1 -> Logical Operator1/1  "LowerLimit_Is_Reached"
  Constant1/1 -> Relational Operator/2
  Constant3/1 -> Relational Operator1/2
  Compare To Zero/1 -> Logical Operator/2  "Error_is_positive"
  Logical Operator/1 -> Logical Operator2/1
  Logical Operator1/1 -> Logical Operator2/2
  Compare To Zero1/1 -> Logical Operator1/2  "Error_is_negative"
  Error/1 -> Compare To Zero1/1, Compare To Zero/1, Product/2, Product1/1
  Sum6/1 -> Saturation2/1
  Product/1 -> Zero-Order Hold/1
  Discrete-Time Integrator/1 -> Sum6/2
  Saturation2/1 -> Out/1
  Switch/1 -> Discrete-Time Integrator/1
  Product1/1 -> Switch/3
  Constant2/1 -> Product/1

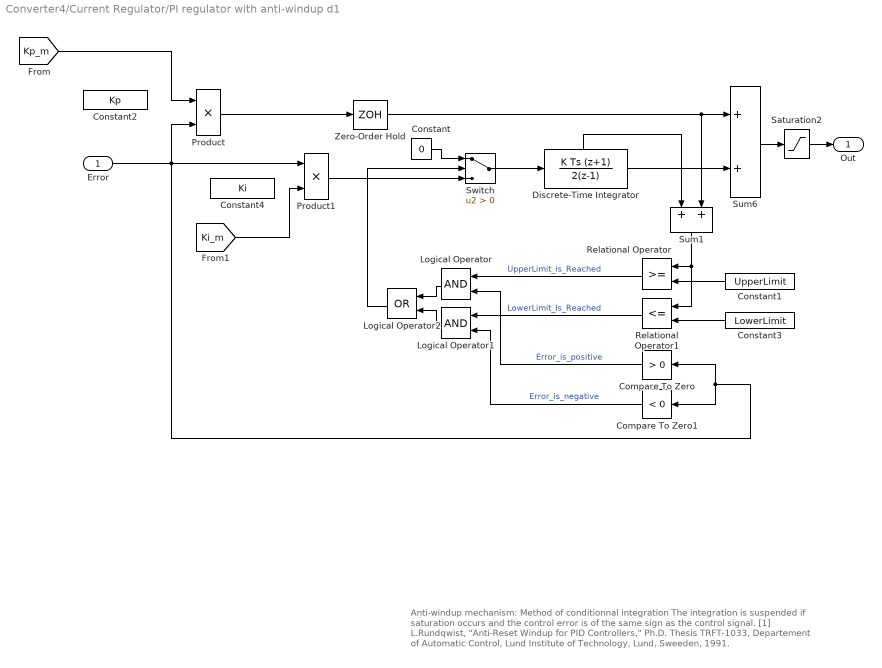
== system Converter4/Current Regulator/PI regulator with anti-windup d1 ==
  note: Anti-windup mechanism: Method of conditionnal integration
      |
      | The integration is suspended if saturation occurs and the
      | control error is of the same sign as the control signal.
      |
      | [1] L.Rundqwist, "Anti-Reset Windup for PID Controllers," Ph.D. Thesis TRFT-1033,
      | Departement of Automatic Control, Lund Institute of Technology, Lund, Sweeden, 1991.
  Error : Inport  SampleTime=Ts
  Compare To Zero : simulink/Logic and Bit Operations/Compare To Zero  relop=>  OutDataTypeStr=uint8  ZeroCross=off
  Compare To Zero1 : simulink/Logic and Bit Operations/Compare To Zero  relop=<  OutDataTypeStr=uint8  ZeroCross=off
  Constant : Constant  Value=0
  Constant1 : Constant  Value=UpperLimit
  Constant2 : Constant  Value=Kp  SampleTime=Ts
  Constant3 : Constant  Value=LowerLimit
  Constant4 : Constant  Value=Ki  SampleTime=Ts
  Discrete-Time Integrator : DiscreteIntegrator  IntegratorMethod=Integration: Trapezoidal  InitialCondition=Init  SampleTime=Ts  LimitOutput=on  UpperSaturationLimit=UpperLimit  LowerSaturationLimit=LowerLimit  ShowStatePort=on  ICPrevOutput=DiscIntNeverNeededParam  ICPrevScaledInput=DiscIntNeverNeededParam
  Logical Operator : Logic  AllPortsSameDT=off  OutDataTypeStr=boolean
  Logical Operator1 : Logic  AllPortsSameDT=off  OutDataTypeStr=boolean
  Logical Operator2 : Logic  Operator=OR  AllPortsSameDT=off  OutDataTypeStr=boolean
  Product : Product
  Product1 : Product
  Relational Operator : RelationalOperator  OutDataTypeStr=boolean  InputSameDT=off
  Relational Operator1 : RelationalOperator  Operator=<=  OutDataTypeStr=boolean  InputSameDT=off
  Saturation2 : Saturate  UpperLimit=UpperLimit  LowerLimit=LowerLimit  SampleTime=Ts
  Sum1 : Sum  InputSameDT=on  SaturateOnIntegerOverflow=on  SampleTime=Ts  OutDataTypeStr=Inherit: Same as first input
  Sum6 : Sum  InputSameDT=on  SaturateOnIntegerOverflow=on  SampleTime=Ts  OutDataTypeStr=Inherit: Same as first input
  Switch : Switch  Criteria=u2 > Threshold  SaturateOnIntegerOverflow=off  InputSameDT=off
  Zero-Order Hold : ZeroOrderHold  SampleTime=Ts
  Out : Outport  SampleTime=Ts  InitialOutput=0  VectorParamsAs1DForOutWhenUnconnected=off
  wires:
  [Ki_m] -> Product1/2
  Constant/1 -> Switch/1
  Zero-Order Hold/1 -> Sum1/2, Sum6/1
  Discrete-Time Integrator/State -> Sum1/1
  Sum1/1 -> Relational Operator1/1, Relational Operator/1
  Logical Operator2/1 -> Switch/2
  Relational Operator/1 -> Logical Operator/1  "UpperLimit_is_Reached"
  Relational Operator1/1 -> Logical Operator1/1  "LowerLimit_Is_Reached"
  Constant1/1 -> Relational Operator/2
  Constant3/1 -> Relational Operator1/2
  Compare To Zero/1 -> Logical Operator/2  "Error_is_positive"
  Logical Operator/1 -> Logical Operator2/1
  Logical Operator1/1 -> Logical Operator2/2
  Compare To Zero1/1 -> Logical Operator1/2  "Error_is_negative"
  Error/1 -> Compare To Zero1/1, Compare To Zero/1, Product/2, Product1/1
  Sum6/1 -> Saturation2/1
  Product/1 -> Zero-Order Hold/1
  Discrete-Time Integrator/1 -> Sum6/2
  Saturation2/1 -> Out/1
  Switch/1 -> Discrete-Time Integrator/1
  Product1/1 -> Switch/3
  [Kp_m] -> Product/1
